simulink model "MLcombiner"  (R2022a)
settings: Solver=FixedStepDiscrete  StartTime=0.0  StopTime=500000  RelTol=1e-3
InitFcn:
  | KCMA = 25;
  | pn11 = GeneratePN11;
  | DetectionFilter = [0.010378066969709
  |    0.023688987704657
  |    0.009767134822858
  |   -0.027017804469398
  |   -0.089762303133391
  |   -0.110346523809347
  |   -0.051853991233850
  |    0.154921158891652
  |    0.568943123186263
  |    0.792392871766106
  |    0.792392871766106
  |    0.568943123186263
  |    0.154921158891652
  |   -0.051853991233850
  |   -0.110346523809347
  |   -0.089762303133391
  |   -0.027017804469398
  |    0.009767134822858
  |    0.023688987704657
  |    0.010378066969709];
  | E1 = h1_pruned'*h1_pruned;
  | E2 = h2_pruned'*h2_pruned;
  | muCMA = 1/((2*KCMA+1)*(E1+E2));
undefined symbols (not defined in the file): h1_pruned, h2_pruned, jsin, pskmod, SOQPSK_frequency_pulse
libraries: dspsrcs4 x5, simulink x3, commeq3 x1, dspmlti4 x1, dspsigops x1
settings Model: Creator=rice  LastModifiedBy=mdr
settings SolverCC: AlgebraicLoopSolver=TrustRegion
settings DebuggingCC: UnconnectedInputMsg=warning  UnconnectedOutputMsg=warning  UnconnectedLineMsg=warning  SFMachineParentedDataDiag=warning  UnderSpecifiedDimensionMsg=warning
settings RTWCC: DLArmComputeVersion=19.05

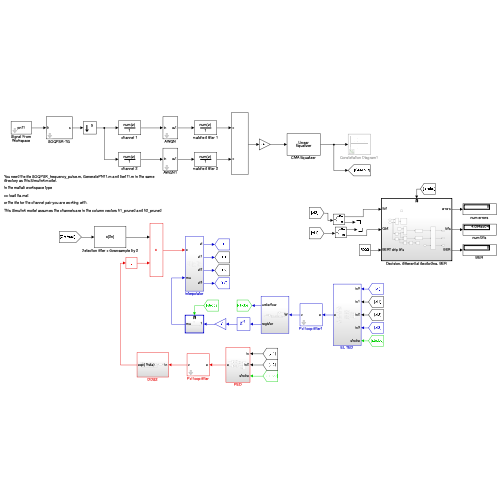
[thumbnail: Simulink's stored preview of the top-level diagram]
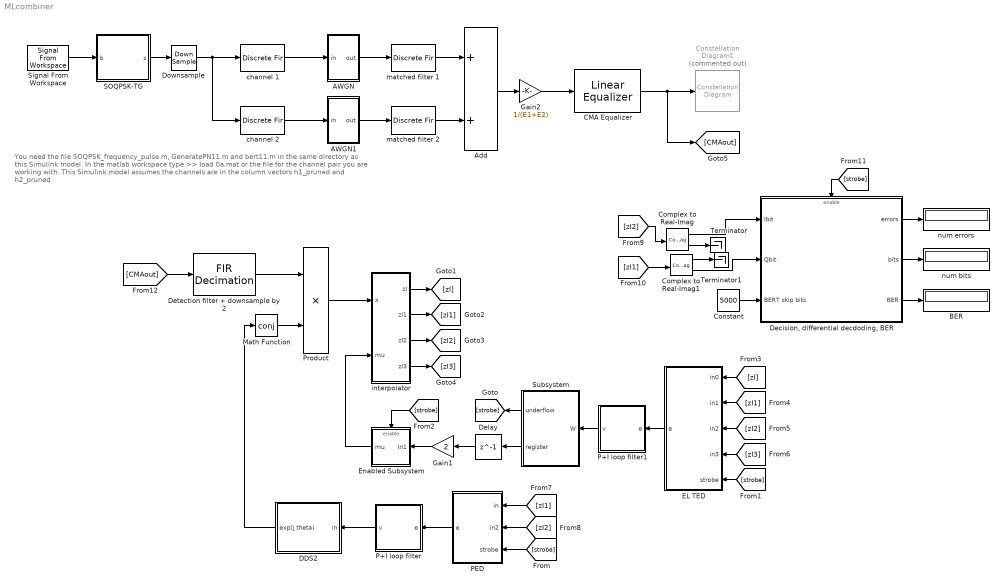
== system MLcombiner ==
  note: You need the file SOQPSK_frequency_pulse.m, GeneratePN11.m and bert11.m in the same directory as this Simulink model.
      |
      | In the matlab workspace type
      |
      | >> load 0a.mat
      |
      | or the file for the channel pair you are working with.
      |
      | This Simulink model assumes the channels are in the column vectors h1_pruned and h2_pruned
  AWGN : Subsystem  mask{N0dB=0}
      mask prompts: N0dB "N0 (dB)"
      mask init:
      | nvar = 10^(0.1*N0dB);
      | nstd = sqrt(nvar);
      | 
      | thisSampleTime = get_param(gcb,'CompiledSampleTime');
  AWGN1 : Subsystem  mask{N0dB=0}
      mask prompts: N0dB "N0 (dB)"
      mask init:
      | nvar = 10^(0.1*N0dB);
      | nstd = sqrt(nvar);
      | 
      | thisSampleTime = get_param(gcb,'CompiledSampleTime');
  Add : Sum
  BER : Display
  CMA Equalizer : commeq3/Linear Equalizer  NumTaps=2*KCMA+1  Constellation=pskmod( 0:3, 4, pi/4 )  InputSamplesPerSymbol=1  Algorithm=CMA  StepSize=muCMA  ForgettingFactor=0.99  InitialInverseCorrelationMatrix=0.1  ReferenceTap=KCMA+1  InputDelay=0  AdaptWeightsSource=Property  AdaptWeights=on  InitialWeightsSource=Auto  InitialWeights=0  TrainingInitialWeights=0  BlindInitialWeights=[ 0; 0; 1; 0; 0 ]  WeightUpdatePeriod=1  TrainingFlagInputPort=off  AdaptAfterTraining=on  ResetInputPort=off  ErrorOutputPort=off  TapWeightsOutputPort=off  SimulateUsing=Code generation
      settings: SourceProductBaseCode=CM
  Complex to Real-Imag : ComplexToRealImag
  Complex to Real-Imag1 : ComplexToRealImag
  Constant : Constant  Value=5000
  Constellation Diagram1 : ConstellationDiagram  Commented=on  WindowPosition=[1688.000000,1144.000000,359.000000,366.000000,]  ScopeFrameLocation=window  SymbolsToDisplaySource=Property  SymbolsToDisplay=400  DefaultConfigurationName=comm.scopes.ConstellationDiagramBlockCfg
  DDS2 : Subsystem
  "Decision, differential decdoding, BER" : Subsystem  TreatAsAtomicUnit=on
  Delay : Delay  DelayLength=1
  Detection filter + downsample by 2 : dspmlti4/FIR Decimation  FilterSource=Dialog parameters  h=DetectionFilter.'  D=2  filtStruct=Direct form  FilterObject=FDECIM  framing=Enforce single-rate processing  inputOffset=0  outputBufInitCond=0  roundingMode=Floor  overflowMode=off  firstCoeffDataTypeStr=Inherit: Same word length as input  firstCoeffMin=[]  firstCoeffMax=[]  firstCoeffLastDataTypeStr=Inherit: Same word length as input  outputDataTypeStr=Inherit: Same as accumulator  outputMin=[]  outputMax=[]  outputLastDataTypeStr=Inherit: Same as accumulator
  Downsample : DownSample  N=5  RateOptions=Allow multirate processing
  EL TED : Subsystem
  Enabled Subsystem : Subsystem  TreatAsAtomicUnit=on
  Gain1 : Gain  Gain=2
  Gain2 : Gain  Gain=1/(E1+E2)
  Math Function : Math  Operator=conj
  P+I loop filter : Subsystem  mask{BnTs=0.01, zeta=1, N=2, Kp=3.9, K0=1}
      mask prompts: BnTs "closed loop bandwidth (BnTs)"; zeta "damping factor"; N "sample rate (samples/symbol)"; Kp "PED gain"; K0 "DDS gain"
      mask init:
      | foo = BnTs/(N*(zeta + 0.25/zeta));
      | d = 1 + 2*zeta*foo + foo*foo;
      | K1 = 4*zeta*foo/(d*K0*Kp);
      | K2 = 4*foo*foo/(d*K0*Kp);
  P+I loop filter1 : Subsystem  mask{BnTs=0.01, zeta=1, N=2, Kp=5.3, K0=-1}
      mask prompts: BnTs "closed loop bandwidth (BnTs)"; zeta "damping factor"; N "sample rate (samples/symbol)"; Kp "PED gain"; K0 "DDS gain"
      mask init:
      | foo = BnTs/(N*(zeta + 0.25/zeta));
      | d = 1 + 2*zeta*foo + foo*foo;
      | K1 = 4*zeta*foo/(d*K0*Kp);
      | K2 = 4*foo*foo/(d*K0*Kp);
  PED : Subsystem
  Product : Product
  SOQPSK-TG : Subsystem  mask{Nb=10}
      mask prompts: Nb "samples/bit"
  Signal From Workspace : dspsrcs4/Signal From Workspace  X=pn11  Ts=1  nsamps=1  OutputAfterFinalValue=Cyclic repetition  ignoreOrWarnInputAndFrameLengths=off  OutputFrames=off
  Subsystem : Subsystem
  Terminator : Terminator
  Terminator1 : Terminator
  channel 1 : DiscreteFir  Coefficients=h1_pruned.'
  channel 2 : DiscreteFir  Coefficients=h2_pruned.'
  interpolator : Subsystem
  matched filter 1 : DiscreteFir  Coefficients=h1_pruned(end:-1:1)'
  matched filter 2 : DiscreteFir  Coefficients=h2_pruned(end:-1:1)'
  num bits : Display
  num errors : Display
  wires:
  CMA Equalizer/1 -> [CMAout], Constellation Diagram1/1
  Math Function/1 -> Product/2
  Detection filter + downsample by 2/1 -> Product/1
  DDS2/1(exp(j theta)) -> Math Function/1
  Product/1 -> interpolator/1(x)
  PED/1(e) -> P+I loop filter/1(e)
  P+I loop filter/1(v) -> DDS2/1(in)
  EL TED/1(e) -> P+I loop filter1/1(e)
  P+I loop filter1/1(v) -> Subsystem/1(W)
  Subsystem/1(underflow) -> [strobe]
  [strobe] -> PED/3(strobe)
  [strobe] -> EL TED/5(strobe)
  Subsystem/2(register) -> Delay/1
  Delay/1 -> Gain1/1
  Gain1/1 -> Enabled Subsystem/1(In1)
  Enabled Subsystem/1(mu) -> interpolator/2(mu)
  [strobe] -> Enabled Subsystem/Enable
  interpolator/1(zI) -> [zI]
  interpolator/4(zI3) -> [zI3]
  interpolator/2(zI1) -> [zI1]
  interpolator/3(zI2) -> [zI2]
  [zI] -> EL TED/1(in0)
  [zI1] -> EL TED/2(in1)
  [zI2] -> EL TED/3(in2)
  [zI3] -> EL TED/4(in3)
  [zI1] -> PED/1(in)
  [zI2] -> PED/2(in2)
  [zI2] -> Complex to Real-Imag/1
  [zI1] -> Complex to Real-Imag1/1
  Complex to Real-Imag/1 -> "Decision, differential decdoding, BER"/1(Ibit)
  Complex to Real-Imag1/2 -> "Decision, differential decdoding, BER"/2(Qbit)
  Complex to Real-Imag/2 -> Terminator/1
  Complex to Real-Imag1/1 -> Terminator1/1
  [strobe] -> "Decision, differential decdoding, BER"/Enable
  "Decision, differential decdoding, BER"/2(bits) -> num bits/1
  "Decision, differential decdoding, BER"/3(BER) -> BER/1
  "Decision, differential decdoding, BER"/1(errors) -> num errors/1
  [CMAout] -> Detection filter + downsample by 2/1
  Constant/1 -> "Decision, differential decdoding, BER"/3(BERT skip bits)
  Signal From Workspace/1 -> SOQPSK-TG/1(b)
  SOQPSK-TG/1(s) -> Downsample/1
  channel 1/1 -> AWGN/1(in)
  channel 2/1 -> AWGN1/1(in)
  AWGN1/1(out) -> matched filter 2/1
  AWGN/1(out) -> matched filter 1/1
  matched filter 1/1 -> Add/1
  matched filter 2/1 -> Add/2
  Downsample/1 -> channel 1/1, channel 2/1
  Add/1 -> Gain2/1
  Gain2/1 -> CMA Equalizer/1

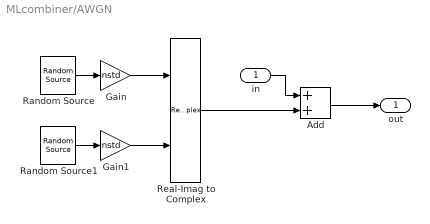
== system MLcombiner/AWGN ==
  in : Inport
  Add : Sum
  Gain : Gain  Gain=nstd
  Gain1 : Gain  Gain=nstd
  Random Source : dspsrcs4/Random Source  SrcType=Gaussian  NormMethod=Ziggurat  CltLength=12  MinVal=0  MaxVal=1  MeanVal=0  VarVal=1  RepMode=Not repeatable  rawSeed=1  IsInherit=off  SampMode=Discrete  SampTime=thisSampleTime(1)  SampFrame=1  DataType=Double  OutComplex=Real  OutputFrames=off
  Random Source1 : dspsrcs4/Random Source  SrcType=Gaussian  NormMethod=Ziggurat  CltLength=12  MinVal=0  MaxVal=1  MeanVal=0  VarVal=1  RepMode=Not repeatable  rawSeed=1  IsInherit=off  SampMode=Discrete  SampTime=thisSampleTime(1)  SampFrame=1  DataType=Double  OutComplex=Real  OutputFrames=off
  Real-Imag to Complex : RealImagToComplex
  out : Outport
  wires:
  Random Source/1 -> Gain/1
  Random Source1/1 -> Gain1/1
  Gain1/1 -> Real-Imag to Complex/2
  Gain/1 -> Real-Imag to Complex/1
  Real-Imag to Complex/1 -> Add/2
  Add/1 -> out/1
  in/1 -> Add/1

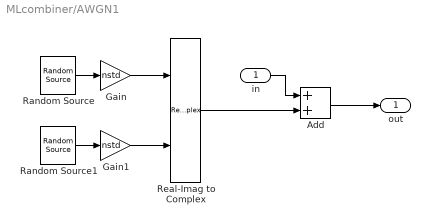
== system MLcombiner/AWGN1 ==
  in : Inport
  Add : Sum
  Gain : Gain  Gain=nstd
  Gain1 : Gain  Gain=nstd
  Random Source : dspsrcs4/Random Source  SrcType=Gaussian  NormMethod=Ziggurat  CltLength=12  MinVal=0  MaxVal=1  MeanVal=0  VarVal=1  RepMode=Not repeatable  rawSeed=1  IsInherit=off  SampMode=Discrete  SampTime=thisSampleTime(1)  SampFrame=1  DataType=Double  OutComplex=Real  OutputFrames=off
  Random Source1 : dspsrcs4/Random Source  SrcType=Gaussian  NormMethod=Ziggurat  CltLength=12  MinVal=0  MaxVal=1  MeanVal=0  VarVal=1  RepMode=Not repeatable  rawSeed=1  IsInherit=off  SampMode=Discrete  SampTime=thisSampleTime(1)  SampFrame=1  DataType=Double  OutComplex=Real  OutputFrames=off
  Real-Imag to Complex : RealImagToComplex
  out : Outport
  wires:
  in/1 -> Add/1
  Add/1 -> out/1
  Real-Imag to Complex/1 -> Add/2
  Gain/1 -> Real-Imag to Complex/1
  Gain1/1 -> Real-Imag to Complex/2
  Random Source1/1 -> Gain1/1
  Random Source/1 -> Gain/1

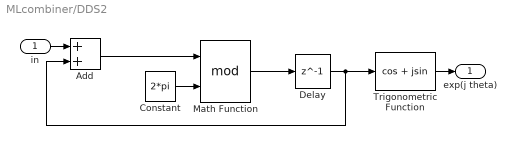
== system MLcombiner/DDS2 ==
  in : Inport
  Add : Sum
  Constant : Constant  Value=2*pi
  Delay : Delay  DelayLength=1
  Math Function : Math  Operator=mod
  Trigonometric Function : Trigonometry  Operator=cos + jsin
  exp(j theta) : Outport
  wires:
  Constant/1 -> Math Function/2
  in/1 -> Add/1
  Trigonometric Function/1 -> exp(j theta)/1
  Math Function/1 -> Delay/1
  Delay/1 -> Add/2, Trigonometric Function/1
  Add/1 -> Math Function/1

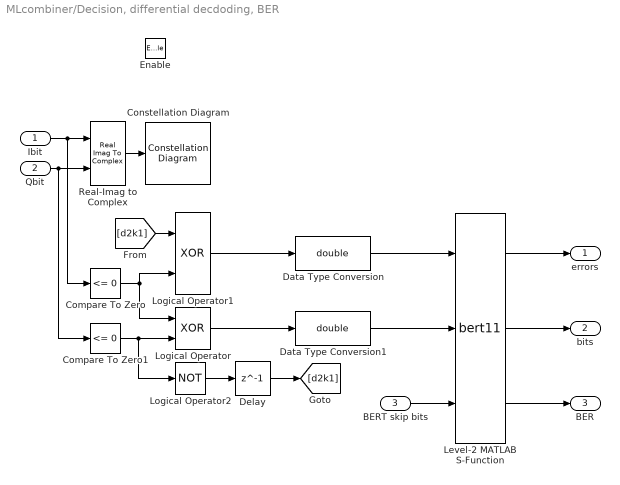
== system MLcombiner/Decision, differential decdoding, BER ==
  Ibit : Inport
  Qbit : Inport  Port=2
  BERT skip bits : Inport  Port=3
  Enable : EnablePort
  Compare To Zero : simulink/Logic and Bit Operations/Compare To Zero  relop=<=  OutDataTypeStr=boolean
  Compare To Zero1 : simulink/Logic and Bit Operations/Compare To Zero  relop=<=  OutDataTypeStr=boolean
  Constellation Diagram : ConstellationDiagram  WindowPosition=[1686.000000,743.000000,359.000000,366.000000,]  Visible=on  ScopeFrameLocation=window  SymbolsToDisplaySource=Property  SymbolsToDisplay=400  ReferenceConstellation="{[2+2i                    -2+2i                    -2-2i                     2-2i]}"  XLimits=[-2.7774 2.6966]  YLimits=[-3.4617 3.3809]  DefaultConfigurationName=comm.scopes.ConstellationDiagramBlockCfg
  Data Type Conversion : DataTypeConversion  OutDataTypeStr=double  SaturateOnIntegerOverflow=off  RndMeth=Floor
  Data Type Conversion1 : DataTypeConversion  OutDataTypeStr=double  SaturateOnIntegerOverflow=off  RndMeth=Floor
  Delay : Delay  DelayLength=1
  Level-2 MATLAB S-Function : M-S-Function  FunctionName=bert11
  Logical Operator : Logic  Operator=XOR  AllPortsSameDT=off  OutDataTypeStr=boolean
  Logical Operator1 : Logic  Operator=XOR  AllPortsSameDT=off  OutDataTypeStr=boolean
  Logical Operator2 : Logic  Operator=NOT  AllPortsSameDT=off  OutDataTypeStr=boolean
  Real-Imag to Complex : RealImagToComplex
  errors : Outport
  bits : Outport  Port=2
  BER : Outport  Port=3
  wires:
  Real-Imag to Complex/1 -> Constellation Diagram/1
  Ibit/1 -> Compare To Zero/1, Real-Imag to Complex/1
  Qbit/1 -> Compare To Zero1/1, Real-Imag to Complex/2
  Compare To Zero1/1 -> Logical Operator2/1, Logical Operator/2
  Compare To Zero/1 -> Logical Operator/1, Logical Operator1/2
  [d2k1] -> Logical Operator1/1
  Delay/1 -> [d2k1]
  Logical Operator2/1 -> Delay/1
  Logical Operator1/1 -> Data Type Conversion/1
  Logical Operator/1 -> Data Type Conversion1/1
  Level-2 MATLAB S-Function/3 -> BER/1
  Level-2 MATLAB S-Function/2 -> bits/1
  Level-2 MATLAB S-Function/1 -> errors/1
  BERT skip bits/1 -> Level-2 MATLAB S-Function/3
  Data Type Conversion/1 -> Level-2 MATLAB S-Function/1
  Data Type Conversion1/1 -> Level-2 MATLAB S-Function/2

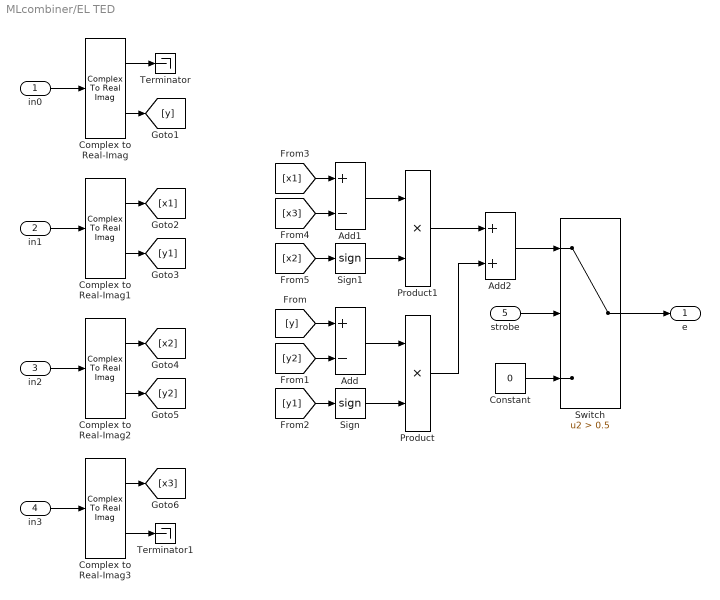
== system MLcombiner/EL TED ==
  in0 : Inport
  in1 : Inport  Port=2
  in2 : Inport  Port=3
  in3 : Inport  Port=4
  strobe : Inport  Port=5
  Add : Sum  Inputs=+-
  Add1 : Sum  Inputs=+-
  Add2 : Sum
  Complex to Real-Imag{,1..3} (4 alike) : ComplexToRealImag
  Constant : Constant  Value=0
  Product : Product
  Product1 : Product
  Sign : Signum
  Sign1 : Signum
  Switch : Switch  Criteria=u2 > Threshold  Threshold=0.5  SaturateOnIntegerOverflow=off  InputSameDT=off
  Terminator : Terminator
  Terminator1 : Terminator
  e : Outport
  wires:
  Complex to Real-Imag/1 -> Terminator/1
  in1/1 -> Complex to Real-Imag1/1
  [y2] -> Add/2
  Complex to Real-Imag3/1 -> [x3]
  Add1/1 -> Product1/1
  Add2/1 -> Switch/1
  Sign1/1 -> Product1/2
  Product1/1 -> Add2/1
  in0/1 -> Complex to Real-Imag/1
  [x3] -> Add1/2
  [x2] -> Sign1/1
  [y] -> Add/1
  in3/1 -> Complex to Real-Imag3/1
  [x1] -> Add1/1
  Product/1 -> Add2/2
  in2/1 -> Complex to Real-Imag2/1
  Complex to Real-Imag/2 -> [y]
  Constant/1 -> Switch/3
  Switch/1 -> e/1
  Sign/1 -> Product/2
  strobe/1 -> Switch/2
  Complex to Real-Imag2/1 -> [x2]
  Complex to Real-Imag1/1 -> [x1]
  Complex to Real-Imag3/2 -> Terminator1/1
  Add/1 -> Product/1
  Complex to Real-Imag2/2 -> [y2]
  [y1] -> Sign/1
  Complex to Real-Imag1/2 -> [y1]

== system MLcombiner/Enabled Subsystem ==
  In1 : Inport
  Enable : EnablePort
  mu : Outport
  wires:
  In1/1 -> mu/1

== system MLcombiner/P+I loop filter ==
  e : Inport
  Discrete Filter : DiscreteFilter  Numerator=[(K1+K2) -K1]  Denominator=[1 -1]
  v : Outport
  wires:
  e/1 -> Discrete Filter/1
  Discrete Filter/1 -> v/1

== system MLcombiner/P+I loop filter1 ==
  e : Inport
  Discrete Filter : DiscreteFilter  Numerator=[(K1+K2) -K1]  Denominator=[1 -1]
  v : Outport
  wires:
  Discrete Filter/1 -> v/1
  e/1 -> Discrete Filter/1

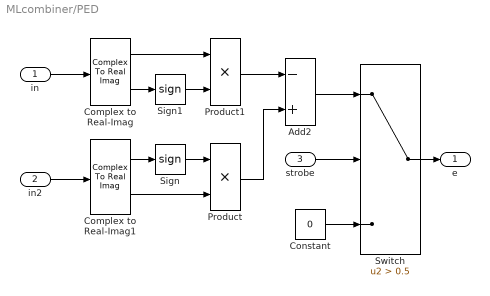
== system MLcombiner/PED ==
  in : Inport
  in2 : Inport  Port=2
  strobe : Inport  Port=3
  Add2 : Sum  Inputs=-+
  Complex to Real-Imag : ComplexToRealImag
  Complex to Real-Imag1 : ComplexToRealImag
  Constant : Constant  Value=0
  Product : Product
  Product1 : Product
  Sign : Signum
  Sign1 : Signum
  Switch : Switch  Criteria=u2 > Threshold  Threshold=0.5  SaturateOnIntegerOverflow=off  InputSameDT=off
  e : Outport
  wires:
  in2/1 -> Complex to Real-Imag1/1
  Constant/1 -> Switch/3
  in/1 -> Complex to Real-Imag/1
  Switch/1 -> e/1
  Product1/1 -> Add2/1
  Product/1 -> Add2/2
  strobe/1 -> Switch/2
  Add2/1 -> Switch/1
  Complex to Real-Imag1/1 -> Sign/1
  Sign/1 -> Product/1
  Complex to Real-Imag1/2 -> Product/2
  Complex to Real-Imag/2 -> Sign1/1
  Sign1/1 -> Product1/2
  Complex to Real-Imag/1 -> Product1/1

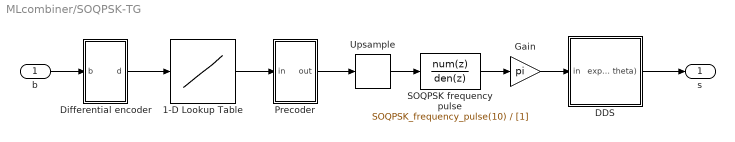
== system MLcombiner/SOQPSK-TG ==
  b : Inport
  1-D Lookup Table : Lookup_n-D  NumberOfTableDimensions=1  BreakpointsForDimension1=[0 1]  Table=[-1 1]  InternalRulePriority=Speed  RndMeth=Simplest
  DDS : Subsystem
  Differential encoder : Subsystem
  Gain : Gain  Gain=pi
  Precoder : Subsystem
  SOQPSK frequency pulse : DiscreteFilter  Numerator=SOQPSK_frequency_pulse(10)  Denominator=[1]
  Upsample : dspsigops/Upsample  N=Nb  phase=0  RateOptions=Allow multirate processing  ic=0  mode=Unused parameter value
  s : Outport
  wires:
  DDS/1(exp(j theta)) -> s/1
  b/1 -> Differential encoder/1(b)
  Precoder/1(out) -> Upsample/1
  Differential encoder/1(d) -> 1-D Lookup Table/1
  Gain/1 -> DDS/1(in)
  Upsample/1 -> SOQPSK frequency pulse/1
  1-D Lookup Table/1 -> Precoder/1(in)
  SOQPSK frequency pulse/1 -> Gain/1

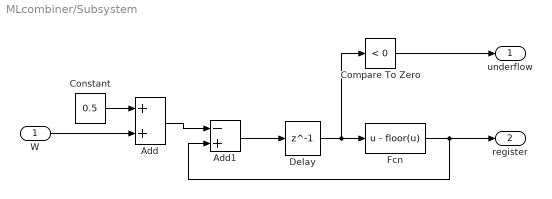
== system MLcombiner/Subsystem ==
  W : Inport
  Add : Sum
  Add1 : Sum  Inputs=-+
  Compare To Zero : simulink/Logic and Bit Operations/Compare To Zero  relop=<  OutDataTypeStr=boolean
  Constant : Constant  Value=0.5
  Delay : Delay  DelayLength=1
  Fcn : Fcn  Expr=u - floor(u)
  underflow : Outport
  register : Outport  Port=2
  wires:
  Compare To Zero/1 -> underflow/1
  W/1 -> Add/2
  Add/1 -> Add1/1
  Add1/1 -> Delay/1
  Constant/1 -> Add/1
  Fcn/1 -> Add1/2, register/1
  Delay/1 -> Compare To Zero/1, Fcn/1

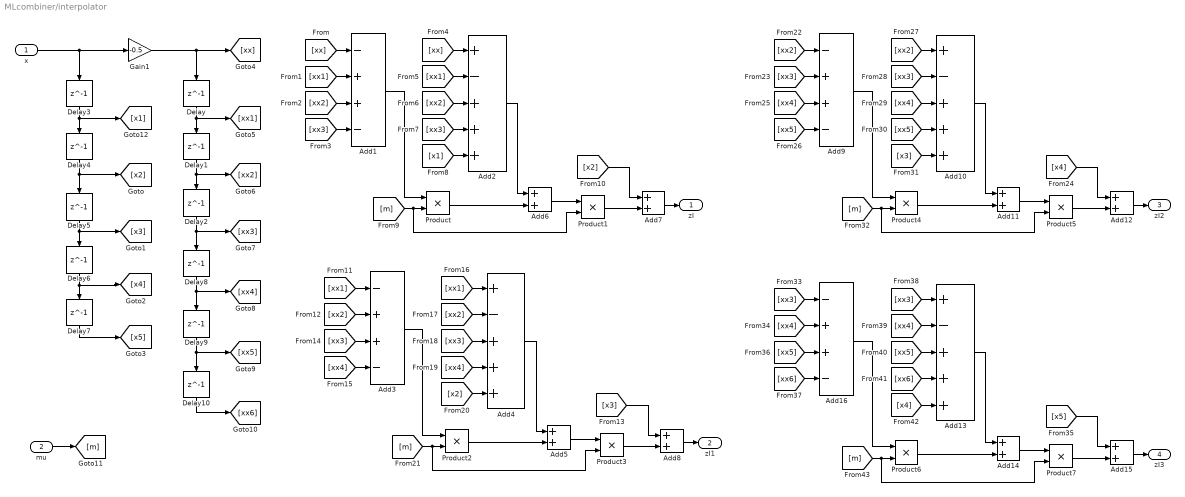
== system MLcombiner/interpolator ==
  x : Inport
  mu : Inport  Port=2
  Add{1,3,9,16} (4 alike) : Sum  Inputs=-++-
  Add{2,4,10,13} (4 alike) : Sum  Inputs=+-+++
  Add{5..8,11..12,14..15} (8 alike) : Sum
  Delay{,1..10} (11 alike) : Delay  DelayLength=1
  Gain1 : Gain  Gain=-0.5
  Product{,1..7} (8 alike) : Product
  zI : Outport
  zI1 : Outport  Port=2
  zI2 : Outport  Port=3
  zI3 : Outport  Port=4
  wires:
  Delay/1 -> Delay1/1, [xx1]
  Add6/1 -> Product1/1
  Add7/1 -> zI/1
  Delay1/1 -> [xx2], Delay2/1
  Product1/1 -> Add7/2
  Delay3/1 -> [x1], Delay4/1
  Product/1 -> Add6/2
  Gain1/1 -> Delay/1, [xx]
  Delay5/1 -> Delay6/1, [x3]
  Delay4/1 -> [x2], Delay5/1
  Delay7/1 -> [x5]
  Delay6/1 -> [x4], Delay7/1
  x/1 -> Delay3/1, Gain1/1
  Delay8/1 -> Delay9/1, [xx4]
  Delay2/1 -> Delay8/1, [xx3]
  Delay9/1 -> Delay10/1, [xx5]
  Delay10/1 -> [xx6]
  mu/1 -> [m]
  [xx] -> Add1/1
  [xx1] -> Add1/2
  [xx2] -> Add1/3
  [xx3] -> Add1/4
  [xx] -> Add2/1
  [xx1] -> Add2/2
  [xx2] -> Add2/3
  [xx3] -> Add2/4
  [x1] -> Add2/5
  Add1/1 -> Product/1
  [m] -> Product1/2, Product/2
  Add2/1 -> Add6/1
  [x2] -> Add7/1
  [x3] -> Add8/1
  Add4/1 -> Add5/1
  [m] -> Product2/2, Product3/2
  Add3/1 -> Product2/1
  [x2] -> Add4/5
  [xx4] -> Add4/4
  [xx3] -> Add4/3
  [xx2] -> Add4/2
  [xx1] -> Add4/1
  [xx4] -> Add3/4
  [xx3] -> Add3/3
  [xx2] -> Add3/2
  [xx1] -> Add3/1
  Product2/1 -> Add5/2
  Product3/1 -> Add8/2
  Add8/1 -> zI1/1
  Add5/1 -> Product3/1
  Add11/1 -> Product5/1
  Add12/1 -> zI2/1
  Product5/1 -> Add12/2
  Product4/1 -> Add11/2
  [xx2] -> Add9/1
  [xx3] -> Add9/2
  [xx4] -> Add9/3
  [xx5] -> Add9/4
  [xx2] -> Add10/1
  [xx3] -> Add10/2
  [xx4] -> Add10/3
  [xx5] -> Add10/4
  [x3] -> Add10/5
  Add9/1 -> Product4/1
  [m] -> Product5/2, Product4/2
  Add10/1 -> Add11/1
  [x4] -> Add12/1
  [x5] -> Add15/1
  Add13/1 -> Add14/1
  [m] -> Product6/2, Product7/2
  Add16/1 -> Product6/1
  [x4] -> Add13/5
  [xx6] -> Add13/4
  [xx5] -> Add13/3
  [xx4] -> Add13/2
  [xx3] -> Add13/1
  [xx6] -> Add16/4
  [xx5] -> Add16/3
  [xx4] -> Add16/2
  [xx3] -> Add16/1
  Product6/1 -> Add14/2
  Product7/1 -> Add15/2
  Add15/1 -> zI3/1
  Add14/1 -> Product7/1

== system MLcombiner/SOQPSK-TG/DDS ==
  in : Inport
  Add : Sum
  Add1 : Sum
  Constant : Constant  Value=3*pi/2 - pi/4
  Delay : Delay  DelayLength=1
  Trigonometric Function : Trigonometry  Operator=cos + jsin
  exp(j theta) : Outport
  wires:
  Delay/1 -> Add1/2, Add/2
  in/1 -> Add/1
  Trigonometric Function/1 -> exp(j theta)/1
  Add/1 -> Delay/1
  Add1/1 -> Trigonometric Function/1
  Constant/1 -> Add1/1

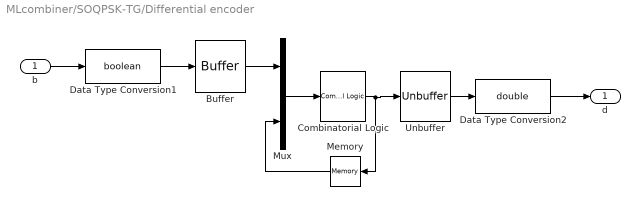
== system MLcombiner/SOQPSK-TG/Differential encoder ==
  b : Inport
  Buffer : Buffer  N=2  OutputFrames=off
  Combinatorial Logic : CombinatorialLogic  TruthTable=[1 1; 0 0; 1 1; 0 0; 1 0; 0 1; 1 0; 0 1; 0 0; 1 1; 0 0; 1 1; 0 1; 1 0; 0 1; 1 0]
  Data Type Conversion1 : DataTypeConversion  OutDataTypeStr=boolean  SaturateOnIntegerOverflow=off  RndMeth=Floor
  Data Type Conversion2 : DataTypeConversion  OutDataTypeStr=double  SaturateOnIntegerOverflow=off  RndMeth=Floor
  Memory : Memory  InheritSampleTime=on
  Mux : Mux  Inputs=2
  Unbuffer : Unbuffer
  d : Outport
  wires:
  b/1 -> Data Type Conversion1/1
  Mux/1 -> Combinatorial Logic/1
  Data Type Conversion1/1 -> Buffer/1
  Data Type Conversion2/1 -> d/1
  Buffer/1 -> Mux/1
  Combinatorial Logic/1 -> Memory/1, Unbuffer/1
  Memory/1 -> Mux/2
  Unbuffer/1 -> Data Type Conversion2/1

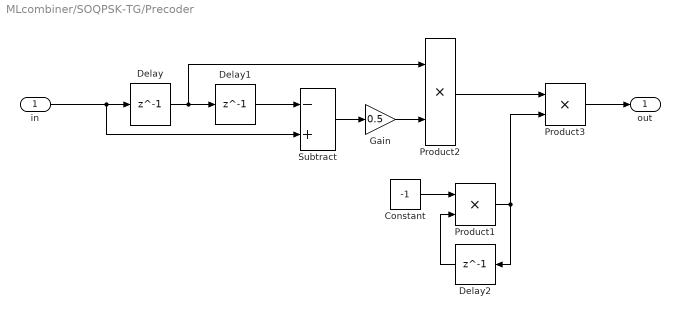
== system MLcombiner/SOQPSK-TG/Precoder ==
  in : Inport
  Constant : Constant  Value=-1
  Delay : Delay  DelayLength=1  InitialCondition=-1  InputProcessing=Columns as channels (frame based)
  Delay1 : Delay  DelayLength=1  InitialCondition=-1  InputProcessing=Columns as channels (frame based)
  Delay2 : Delay  DelayLength=1  InitialCondition=1
  Gain : Gain  Gain=0.5
  Product1 : Product
  Product2 : Product
  Product3 : Product
  Subtract : Sum  Inputs=-+
  out : Outport
  wires:
  Subtract/1 -> Gain/1
  Product2/1 -> Product3/1
  Delay1/1 -> Subtract/1
  Gain/1 -> Product2/2
  in/1 -> Subtract/2, Delay/1
  Delay/1 -> Product2/1, Delay1/1
  Constant/1 -> Product1/1
  Product1/1 -> Product3/2, Delay2/1
  Delay2/1 -> Product1/2
  Product3/1 -> out/1
